simulink model "Induction_motor"  (R2024a)
settings: Solver=VariableStepAuto  StartTime=0.0  StopTime=10  RelTol=1e-3
undefined symbols (not defined in the file or in its folder): x
libraries: spsThreePhaseBreakerLib x6, spsThreePhaseParallelRLCBranchLib x4, spsACVoltageSourceLib x3, POWER_FACTOR x2, spsPower3phInstantaneousLib x2, spsThreePhaseVIMeasurementLib x2, spsAsynchronousMachineSIUnitsLib x1, spsGroundLib x1, Over_Current_Protection_Relay x1, Over_Voltage_Protection_Relay x1, simulink_extras x1, simulink x1
settings Model: Creator=gshma  LastModifiedBy=gshma

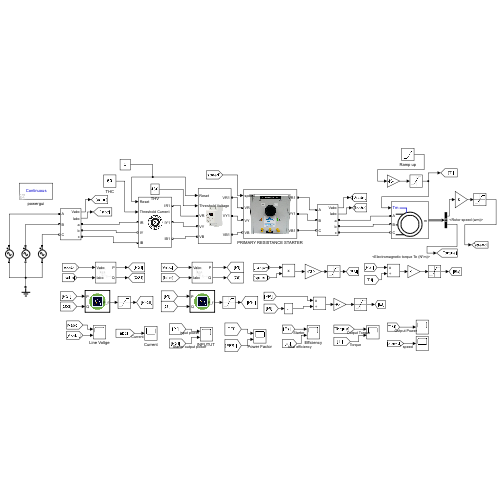
[thumbnail: Simulink's stored preview of the top-level diagram]
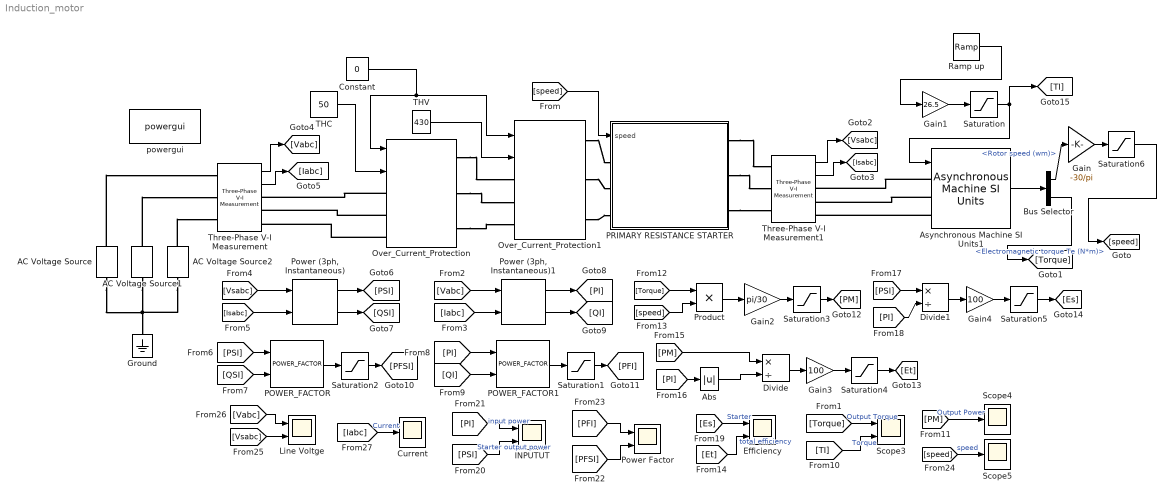
== system Induction_motor ==
  AC Voltage Source : spsACVoltageSourceLib/AC Voltage Source  Amplitude=x/sqrt(3)  Phase=0  Frequency=50  SampleTime=0  Measurements=None  BusType=swing  Pref=10e3  Qref=0  Qmin=-inf  Qmax=+inf
  AC Voltage Source1 : spsACVoltageSourceLib/AC Voltage Source  Amplitude=x/sqrt(3)  Phase=120  Frequency=50  SampleTime=0  Measurements=None  BusType=swing  Pref=10e3  Qref=0  Qmin=-inf  Qmax=+inf
  AC Voltage Source2 : spsACVoltageSourceLib/AC Voltage Source  Amplitude=x/sqrt(3)  Phase=240  Frequency=50  SampleTime=0  Measurements=None  BusType=swing  Pref=10e3  Qref=0  Qmin=-inf  Qmax=+inf
  Abs : Abs  SaturateOnIntegerOverflow=off
  Asynchronous Machine SI Units1 : spsAsynchronousMachineSIUnitsLib/Asynchronous Machine SI Units  RotorType=Squirrel-cage  PresetModel="15:  5.4 HP (4KW)   400 V  50Hz 1430 RPM"  MechanicalLoad=Torque Tm  ShowDetailedParameters=on  ReferenceFrame=Rotor  Units=SI  MeasurementBus=off  NominalParameters=[4000 400 50]  VoltageRatio=1  Stator=[1.405 0.005839]  Rotor=[1.395 0.005839]  Cage1=[0.4155 0.002066]  Cage2=[0.4168 0.0003495]  Lm=0.1722  Mechanical=[0.0131 0.002985 2]  PolePairs=2  InitialConditions=[0.05 0 0 0 0 0 0 0]  SimulateSaturation=off  Saturation=[14.03593122, 27.81365428, 53.79336849, 72.68890987, 97.98006896, 148.6815601, 215.7428561, 302.9841135, 428.7778367 ; 230, 322, 414, 460, 506, 552, 598, 644, 690]  LoadFlowParameters=1492000  TsPowergui=0  TsBlock=-1  IterativeModel=Trapezoidal non iterative  IterativeDiscreteModel=Trapezoidal non iterative  Pmec=1.492e+006
  Bus Selector : BusSelector  OutputSignals=Mechanical.Rotor speed (wm),Mechanical.Electromagnetic torque Te (N*m)
  Constant : Constant  Value=0  OutDataTypeStr=boolean
  Current : Scope
  Divide : Product  Inputs=*/
  Divide1 : Product  Inputs=*/
  Efficiency : Scope  NumInputPorts=2
  Gain : Gain  Gain=-30/pi
  Gain1 : Gain  Gain=26.5
  Gain2 : Gain  Gain=pi/30
  Gain3 : Gain  Gain=100
  Gain4 : Gain  Gain=100
  Ground : spsGroundLib/Ground  LConnTagsString=a
  "INPUTUT " : Scope  NumInputPorts=2
  Line Voltge : Scope  NumInputPorts=2
  Over_Current_Protection : Over_Current_Protection_Relay/Over_Current_Protection  SystemSampleTime=-1  VariantActivationTime=update diagram  AllowFlexibleInterface=on  Latency=0  AutoFrameSizeCalculation=off
  Over_Current_Protection1 : Over_Voltage_Protection_Relay/Over_Current_Protection  SystemSampleTime=-1  VariantActivationTime=update diagram  AllowFlexibleInterface=on  Latency=0  AutoFrameSizeCalculation=off
  POWER_FACTOR : POWER_FACTOR/POWER_FACTOR  SystemSampleTime=-1  VariantActivationTime=update diagram  AllowFlexibleInterface=on  Latency=0  AutoFrameSizeCalculation=off
  POWER_FACTOR1 : POWER_FACTOR/POWER_FACTOR  SystemSampleTime=-1  VariantActivationTime=update diagram  AllowFlexibleInterface=on  Latency=0  AutoFrameSizeCalculation=off
  PRIMARY RESISTANCE STARTER : Subsystem
      mask Display: image('pems.png', [0,0,0,0,80,80]);
  "Power (3ph, Instantaneous)" : spsPower3phInstantaneousLib/Power (3ph, Instantaneous)
  "Power (3ph, Instantaneous)1" : spsPower3phInstantaneousLib/Power (3ph, Instantaneous)
  Power Factor : Scope  NumInputPorts=2
  Product : Product
  Ramp up : simulink/Sources/Ramp  slope=1  start=1  InitialOutput=0
  Saturation : Saturate  UpperLimit=0  LowerLimit=0
  Saturation1 : Saturate  UpperLimit=1  LowerLimit=-1
  Saturation2 : Saturate  UpperLimit=1  LowerLimit=-1
  Saturation3 : Saturate  UpperLimit=4100  LowerLimit=-4000
  Saturation4 : Saturate  UpperLimit=100  LowerLimit=0
  Saturation5 : Saturate  UpperLimit=100  LowerLimit=0
  Saturation6 : Saturate  UpperLimit=2000  LowerLimit=-2000
  Scope3 : Scope  NumInputPorts=2
  Scope4 : Scope
  Scope5 : Scope
  THC : Constant  Value=50
  THV : Constant  Value=430
  Three-Phase V-I Measurement : spsThreePhaseVIMeasurementLib/Three-Phase V-I Measurement  VoltageMeasurement=phase-to-phase  SetLabelV=off  LabelV=Vabc  Vpu=off  VpuLL=off  CurrentMeasurement=yes  SetLabelI=off  LabelI=Iabc  Ipu=off  Pbase=100e6  Vbase=500e3  OutputType=Complex  PhasorSimulation=off  PSBequivalent=0
  Three-Phase V-I Measurement1 : spsThreePhaseVIMeasurementLib/Three-Phase V-I Measurement  VoltageMeasurement=phase-to-phase  SetLabelV=off  LabelV=Vabc  Vpu=off  VpuLL=off  CurrentMeasurement=yes  SetLabelI=off  LabelI=Iabc  Ipu=off  Pbase=100e6  Vbase=500e3  OutputType=Complex  PhasorSimulation=off  PSBequivalent=0
  powergui : sps_lib/powergui  Priority=1  SimulationMode=Continuous  SampleTime=50e-6  frequency=60  Iterations=50  frequencyindice=50  Pbase=100e6  ErrMax=1e-4  UnitsV=kV  UnitsW=MW  buscounter=0  FunctionMessages=off  echomessages=off  EnableUseOfTLC=off  CurrentSourceSwitches=off  DisableSnubberDevices=off  DisableRonSwitches=off  DisableVfSwitches=off  DisplayEquations=off  AutomaticDiscreteSolvers=off  SolverType=Tustin/Backward Euler (TBE)  Interpol=off  ExternalGateDelay=off  methode=off  Ts=100  x0status=blocks  SPID=on  SwTol=0  HookPort=off  NonlinearTolerance=1e-4  nMaxIteration=100  ContinueOnMaxIteration=off  RestoreLinks=warning  ResistiveCurrentMeasurement=off  Frange=[0:2:500]  Ylog=off  Xlog=on  ShowGrid=off  save=off  variable=ZData  structure=0  ZoomFFT=off  StartTime=0.0  cycles=1  DisplayStyle=1  fundamental=60  FreqAxis=off  MaxFrequency=1000  frequencyindicesteady=1  RmsSteady=1  display=off
  wires:
  Asynchronous Machine SI Units1/1 -> Bus Selector/1
  Bus Selector/1 -> Gain/1  "<Rotor speed (wm)>"
  Ramp up/1 -> Gain1/1
  Gain1/1 -> Saturation/1
  [speed] -> PRIMARY RESISTANCE STARTER/1(speed)
  Constant/1 -> Over_Current_Protection/1, Over_Current_Protection1/1
  Saturation/1 -> Asynchronous Machine SI Units1/1, [TI]
  Bus Selector/2 -> [Torque]  "<Electromagnetic torque Te (N*m)>"
  Three-Phase V-I Measurement1/2 -> [Isabc]
  Three-Phase V-I Measurement1/1 -> [Vsabc]
  Three-Phase V-I Measurement/1 -> [Vabc]
  Three-Phase V-I Measurement/2 -> [Iabc]
  THC/1 -> Over_Current_Protection/2
  THV/1 -> Over_Current_Protection1/2
  [Vsabc] -> "Power (3ph, Instantaneous)"/1
  [Isabc] -> "Power (3ph, Instantaneous)"/2
  [Vabc] -> "Power (3ph, Instantaneous)1"/1
  [Iabc] -> "Power (3ph, Instantaneous)1"/2
  "Power (3ph, Instantaneous)"/1 -> [PSI]
  "Power (3ph, Instantaneous)"/2 -> [QSI]
  "Power (3ph, Instantaneous)1"/2 -> [QI]
  "Power (3ph, Instantaneous)1"/1 -> [PI]
  [PSI] -> POWER_FACTOR/1
  [QSI] -> POWER_FACTOR/2
  [PI] -> POWER_FACTOR1/1
  [QI] -> POWER_FACTOR1/2
  POWER_FACTOR1/1 -> Saturation1/1
  Saturation1/1 -> [PFI]
  POWER_FACTOR/1 -> Saturation2/1
  Saturation2/1 -> [PFSI]
  [Torque] -> Product/1
  [speed] -> Product/2
  Product/1 -> Gain2/1
  Gain2/1 -> Saturation3/1
  Saturation3/1 -> [PM]
  [PI] -> Abs/1
  Divide/1 -> Gain3/1
  Gain3/1 -> Saturation4/1
  Saturation4/1 -> [Et]
  Saturation5/1 -> [Es]
  Gain4/1 -> Saturation5/1
  Divide1/1 -> Gain4/1
  [PSI] -> Divide1/1
  [PI] -> Divide1/2
  [PI] -> "INPUTUT "/1  "input power"
  [PSI] -> "INPUTUT "/2  "Starter output power"
  Gain/1 -> Saturation6/1
  Saturation6/1 -> [speed]
  [PFI] -> Power Factor/1
  [PFSI] -> Power Factor/2
  [Es] -> Efficiency/1  "Starter"
  [Et] -> Efficiency/2  "total efficiency"
  [Torque] -> Scope3/1  "Output Torque"
  [TI] -> Scope3/2  "Torque"
  [PM] -> Scope4/1  "Output Power"
  [speed] -> Scope5/1  "speed"
  [Iabc] -> Current/1  "Current"
  Abs/1 -> Divide/2
  [PM] -> Divide/1
  [Vabc] -> Line Voltge/1
  [Vsabc] -> Line Voltge/2
  connections:
  AC Voltage Source/RConn1 -- Three-Phase V-I Measurement/LConn1
  AC Voltage Source1/RConn1 -- Three-Phase V-I Measurement/LConn2
  AC Voltage Source2/RConn1 -- Three-Phase V-I Measurement/LConn3
  AC Voltage Source/LConn1 -- AC Voltage Source2/LConn1 -- Ground/LConn1 -- AC Voltage Source1/LConn1
  Asynchronous Machine SI Units1/LConn1 -- Three-Phase V-I Measurement1/RConn1
  Asynchronous Machine SI Units1/LConn2 -- Three-Phase V-I Measurement1/RConn2
  Asynchronous Machine SI Units1/LConn3 -- Three-Phase V-I Measurement1/RConn3
  PRIMARY RESISTANCE STARTER/RConn1 -- Three-Phase V-I Measurement1/LConn1
  PRIMARY RESISTANCE STARTER/RConn2 -- Three-Phase V-I Measurement1/LConn2
  PRIMARY RESISTANCE STARTER/RConn3 -- Three-Phase V-I Measurement1/LConn3
  Over_Current_Protection/LConn1 -- Three-Phase V-I Measurement/RConn1
  Over_Current_Protection/LConn2 -- Three-Phase V-I Measurement/RConn2
  Over_Current_Protection/LConn3 -- Three-Phase V-I Measurement/RConn3
  Over_Current_Protection/RConn1 -- Over_Current_Protection1/LConn1
  Over_Current_Protection/RConn2 -- Over_Current_Protection1/LConn2
  Over_Current_Protection/RConn3 -- Over_Current_Protection1/LConn3
  Over_Current_Protection1/RConn1 -- PRIMARY RESISTANCE STARTER/LConn1
  Over_Current_Protection1/RConn2 -- PRIMARY RESISTANCE STARTER/LConn2
  Over_Current_Protection1/RConn3 -- PRIMARY RESISTANCE STARTER/LConn3

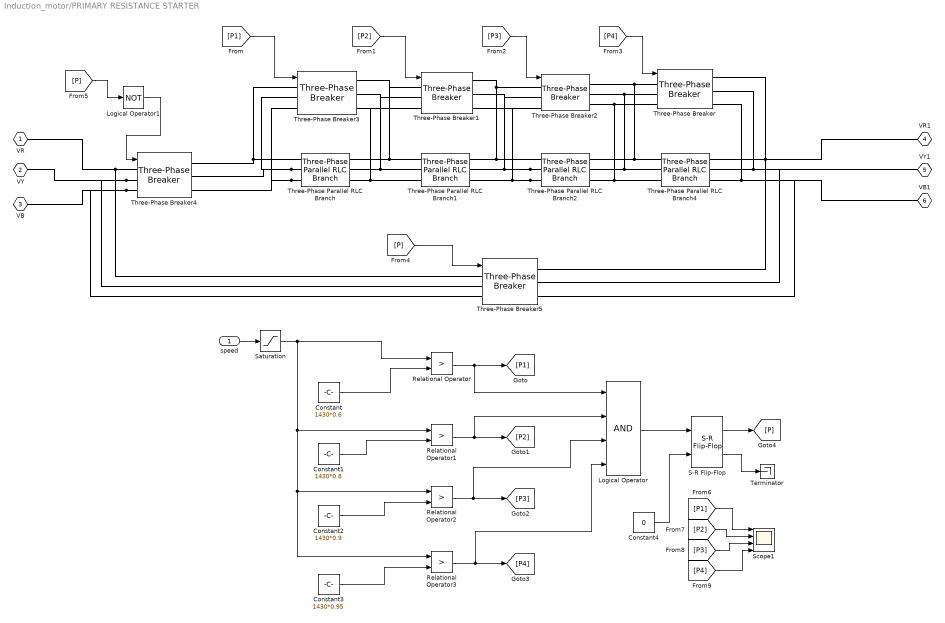
== system Induction_motor/PRIMARY RESISTANCE STARTER ==
  speed : Inport
  Constant : Constant  Value=1430*0.6
  Constant1 : Constant  Value=1430*0.8
  Constant2 : Constant  Value=1430*0.9
  Constant3 : Constant  Value=1430*0.95
  Constant4 : Constant  Value=0  OutDataTypeStr=boolean
  Logical Operator : Logic  Inputs=4  AllPortsSameDT=off  OutDataTypeStr=boolean
  Logical Operator1 : Logic  Operator=NOT  AllPortsSameDT=off  OutDataTypeStr=boolean
  Relational Operator{,1..3} (4 alike) : RelationalOperator  Operator=>  OutDataTypeStr=boolean  RndMeth=Simplest  InputSameDT=off
  S-R Flip-Flop : simulink_extras/Flip Flops/S-R Flip-Flop  initial_condition=0
  Saturation : Saturate  UpperLimit=2000  LowerLimit=0
  Scope1 : Scope  NumInputPorts=4
  Terminator : Terminator
  Three-Phase Parallel RLC Branch{,1..2,4} (4 alike) : spsThreePhaseParallelRLCBranchLib/Three-Phase Parallel RLC Branch  LConnTagsString=A|B|C  RConnTagsString=A|B|C  BranchType=R  Resistance=0.8333  Inductance=1e-3  Capacitance=1e-6  Measurements=None
  Three-Phase Breaker{,1..3,5} (5 alike) : spsThreePhaseBreakerLib/Three-Phase Breaker  InitialState=open  SwitchA=on  SwitchB=on  SwitchC=on  SwitchTimes="[1/60  5/60]"  External=on  BreakerResistance=0.01  SnubberResistance=1e6  SnubberCapacitance=inf  Measurements=None
  Three-Phase Breaker4 : spsThreePhaseBreakerLib/Three-Phase Breaker  InitialState=closed  SwitchA=on  SwitchB=on  SwitchC=on  SwitchTimes="[1/60  5/60]"  External=on  BreakerResistance=0.01  SnubberResistance=1e6  SnubberCapacitance=inf  Measurements=None
  VR : PMIOPort  Tag=simrfV2util1/Connection Port  Side=Left
  VY : PMIOPort  Tag=simrfV2util1/Connection Port  Port=2  Side=Left
  VB : PMIOPort  Tag=simrfV2util1/Connection Port  Port=3  Side=Left
  VR1 : PMIOPort  Tag=simrfV2util1/Connection Port  Port=4  Side=Right
  VY1 : PMIOPort  Tag=simrfV2util1/Connection Port  Port=5  Side=Right
  VB1 : PMIOPort  Tag=simrfV2util1/Connection Port  Port=6  Side=Right
  wires:
  Constant/1 -> Relational Operator/2
  Relational Operator/1 -> Logical Operator/1, [P1]
  speed/1 -> Saturation/1
  Relational Operator1/1 -> Logical Operator/2, [P2]
  Constant1/1 -> Relational Operator1/2
  Constant2/1 -> Relational Operator2/2
  Relational Operator2/1 -> Logical Operator/3, [P3]
  Saturation/1 -> Relational Operator3/1, Relational Operator2/1, Relational Operator1/1, Relational Operator/1
  Relational Operator3/1 -> Logical Operator/4, [P4]
  Constant3/1 -> Relational Operator3/2
  [P1] -> Three-Phase Breaker3/1
  [P2] -> Three-Phase Breaker1/1
  [P3] -> Three-Phase Breaker2/1
  [P4] -> Three-Phase Breaker/1
  [P] -> Three-Phase Breaker5/1
  [P] -> Logical Operator1/1
  Logical Operator1/1 -> Three-Phase Breaker4/1
  Logical Operator/1 -> S-R Flip-Flop/1
  S-R Flip-Flop/1 -> [P]
  S-R Flip-Flop/2 -> Terminator/1
  Constant4/1 -> S-R Flip-Flop/2
  [P1] -> Scope1/1
  [P2] -> Scope1/2
  [P3] -> Scope1/3
  [P4] -> Scope1/4
  connections:
  Three-Phase Parallel RLC Branch/RConn1 -- Three-Phase Parallel RLC Branch1/LConn1 -- Three-Phase Breaker3/RConn1 -- Three-Phase Breaker1/LConn1
  Three-Phase Parallel RLC Branch/RConn2 -- Three-Phase Parallel RLC Branch1/LConn2 -- Three-Phase Breaker3/RConn2 -- Three-Phase Breaker1/LConn2
  Three-Phase Parallel RLC Branch/RConn3 -- Three-Phase Parallel RLC Branch1/LConn3 -- Three-Phase Breaker3/RConn3 -- Three-Phase Breaker1/LConn3
  Three-Phase Breaker1/RConn1 -- Three-Phase Parallel RLC Branch2/LConn1 -- Three-Phase Parallel RLC Branch1/RConn1 -- Three-Phase Breaker2/LConn1
  Three-Phase Parallel RLC Branch2/LConn2 -- Three-Phase Parallel RLC Branch1/RConn2 -- Three-Phase Breaker1/RConn2 -- Three-Phase Breaker2/LConn2
  Three-Phase Parallel RLC Branch2/LConn3 -- Three-Phase Parallel RLC Branch1/RConn3 -- Three-Phase Breaker1/RConn3 -- Three-Phase Breaker2/LConn3
  Three-Phase Breaker2/RConn1 -- Three-Phase Parallel RLC Branch2/RConn1 -- Three-Phase Parallel RLC Branch4/LConn1 -- Three-Phase Breaker/LConn1
  Three-Phase Breaker2/RConn2 -- Three-Phase Parallel RLC Branch2/RConn2 -- Three-Phase Parallel RLC Branch4/LConn2 -- Three-Phase Breaker/LConn2
  Three-Phase Breaker2/RConn3 -- Three-Phase Parallel RLC Branch4/LConn3 -- Three-Phase Parallel RLC Branch2/RConn3 -- Three-Phase Breaker/LConn3
  Three-Phase Breaker3/LConn1 -- Three-Phase Parallel RLC Branch/LConn1 -- Three-Phase Breaker4/RConn1
  Three-Phase Parallel RLC Branch/LConn2 -- Three-Phase Breaker3/LConn2 -- Three-Phase Breaker4/RConn2
  Three-Phase Parallel RLC Branch/LConn3 -- Three-Phase Breaker3/LConn3 -- Three-Phase Breaker4/RConn3
  Three-Phase Breaker/RConn1 -- Three-Phase Parallel RLC Branch4/RConn1 -- VR1/RConn1 -- Three-Phase Breaker5/RConn1
  Three-Phase Breaker/RConn2 -- Three-Phase Parallel RLC Branch4/RConn2 -- VY1/RConn1 -- Three-Phase Breaker5/RConn2
  Three-Phase Breaker/RConn3 -- Three-Phase Parallel RLC Branch4/RConn3 -- Three-Phase Breaker5/RConn3 -- VB1/RConn1
  VR/RConn1 -- Three-Phase Breaker4/LConn1 -- Three-Phase Breaker5/LConn1
  Three-Phase Breaker4/LConn2 -- VY/RConn1 -- Three-Phase Breaker5/LConn2
  Three-Phase Breaker4/LConn3 -- VB/RConn1 -- Three-Phase Breaker5/LConn3
